simulink model "task_2_sim"  (R2023a)
settings: Solver=VariableStepAuto  StartTime=0.0  StopTime=6  MaxStep=1e-4  RelTol=1e-4
undefined symbols (not defined in the file): Ab, Bb, Cb, Cz, D, Dz, Kb, L, xw0, Y1, Y2, Yg
settings Model: Creator=user  LastModifiedBy=user

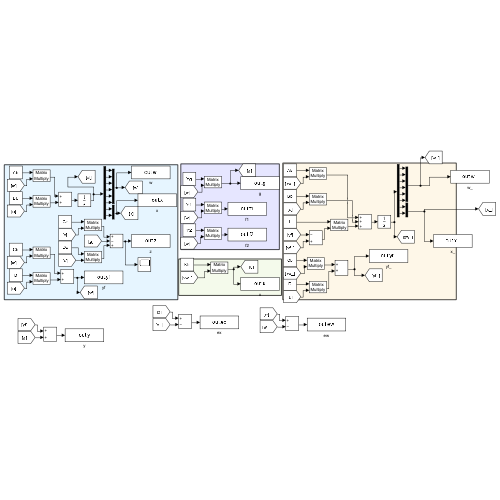
[thumbnail: Simulink's stored preview of the top-level diagram]
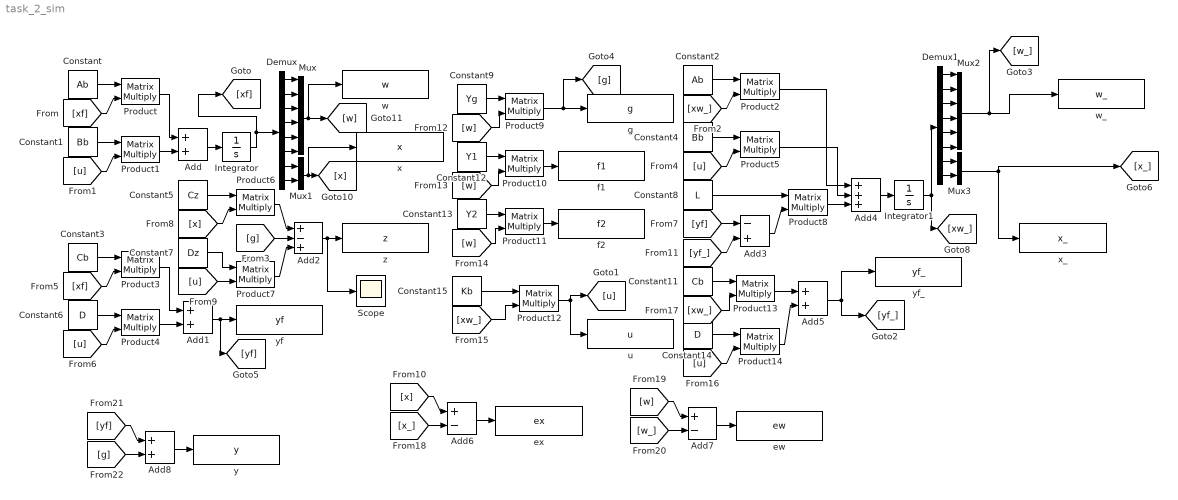
== system task_2_sim ==
  Add{,1,5,8} (4 alike) : Sum
  Add2 : Sum  Inputs=+-+
  Add3 : Sum  Inputs=-+
  Add4 : Sum  Inputs=+++
  Add6 : Sum  Inputs=+-
  Add7 : Sum  Inputs=+-
  Constant : Constant  Value=Ab  VectorParams1D=off
  Constant1 : Constant  Value=Bb  VectorParams1D=off
  Constant11 : Constant  Value=Cb  VectorParams1D=off
  Constant12 : Constant  Value=Y1  VectorParams1D=off
  Constant13 : Constant  Value=Y2  VectorParams1D=off
  Constant14 : Constant  Value=D  VectorParams1D=off
  Constant15 : Constant  Value=Kb  VectorParams1D=off
  Constant2 : Constant  Value=Ab  VectorParams1D=off
  Constant3 : Constant  Value=Cb  VectorParams1D=off
  Constant4 : Constant  Value=Bb  VectorParams1D=off
  Constant5 : Constant  Value=Cz  VectorParams1D=off
  Constant6 : Constant  Value=D  VectorParams1D=off
  Constant7 : Constant  Value=Dz  VectorParams1D=off
  Constant8 : Constant  Value=L  VectorParams1D=off
  Constant9 : Constant  Value=Yg  VectorParams1D=off
  Demux : Demux  Outputs=8
  Demux1 : Demux  Outputs=8
  Integrator : Integrator  InitialCondition=xw0
  Integrator1 : Integrator
  Mux : Mux  Inputs=6
  Mux1 : Mux  Inputs=2
  Mux2 : Mux  Inputs=6
  Mux3 : Mux  Inputs=2
  Product{,1..14} (15 alike) : Product  Multiplication=Matrix(*)
  Scope : Scope
  ew : ToWorkspace  VariableName=ew  SaveFormat=Timeseries  SampleTime=-1
  ex : ToWorkspace  VariableName=ex  SaveFormat=Timeseries  SampleTime=-1
  f1 : ToWorkspace  VariableName=f1  SaveFormat=Timeseries  SampleTime=-1
  f2 : ToWorkspace  VariableName=f2  SaveFormat=Timeseries  SampleTime=-1
  g : ToWorkspace  VariableName=g  SaveFormat=Timeseries  SampleTime=-1
  u : ToWorkspace  VariableName=u  SaveFormat=Timeseries  SampleTime=-1
  w : ToWorkspace  VariableName=w  SaveFormat=Timeseries  SampleTime=-1
  w_ : ToWorkspace  VariableName=w_  SaveFormat=Timeseries  SampleTime=-1
  x : ToWorkspace  VariableName=x  SaveFormat=Timeseries  SampleTime=-1
  x_ : ToWorkspace  VariableName=x_  SaveFormat=Timeseries  SampleTime=-1
  y : ToWorkspace  VariableName=y  SaveFormat=Timeseries  SampleTime=-1
  yf : ToWorkspace  VariableName=yf  SaveFormat=Timeseries  SampleTime=-1
  yf_ : ToWorkspace  VariableName=yf_  SaveFormat=Timeseries  SampleTime=-1
  z : ToWorkspace  VariableName=z  SaveFormat=Timeseries  SampleTime=-1
  wires:
  Constant/1 -> Product/1
  [xf] -> Product/2
  Constant1/1 -> Product1/1
  [u] -> Product1/2
  Constant3/1 -> Product3/1
  [xf] -> Product3/2
  Constant6/1 -> Product4/1
  [u] -> Product4/2
  Product4/1 -> Add1/2
  Product1/1 -> Add/2
  Product3/1 -> Add1/1
  Product/1 -> Add/1
  Add/1 -> Integrator/1
  Integrator/1 -> Demux/1, [xf]
  Add1/1 -> [yf], yf/1
  Constant5/1 -> Product6/1
  [x] -> Product6/2
  [u] -> Product7/2
  Constant7/1 -> Product7/1
  [g] -> Add2/2
  Product7/1 -> Add2/3
  Product6/1 -> Add2/1
  Add2/1 -> Scope/1, z/1
  Constant9/1 -> Product9/1
  [w] -> Product9/2
  Product9/1 -> g/1, [g]
  [w] -> Product10/2
  Constant12/1 -> Product10/1
  Product10/1 -> f1/1
  Constant13/1 -> Product11/1
  [w] -> Product11/2
  Product11/1 -> f2/1
  Constant15/1 -> Product12/1
  [xw_] -> Product12/2
  Product12/1 -> u/1, [u]
  Demux/1 -> Mux/1
  Demux/2 -> Mux/2
  Demux/3 -> Mux/3
  Demux/4 -> Mux/4
  Demux/5 -> Mux/5
  Demux/6 -> Mux/6
  Demux/7 -> Mux1/1
  Demux/8 -> Mux1/2
  Mux1/1 -> x/1, [x]
  Mux/1 -> w/1, [w]
  Constant2/1 -> Product2/1
  [xw_] -> Product2/2
  Constant4/1 -> Product5/1
  [u] -> Product5/2
  [yf_] -> Add3/2
  [yf] -> Add3/1
  Constant8/1 -> Product8/1
  Add3/1 -> Product8/2
  Product8/1 -> Add4/3
  Product5/1 -> Add4/2
  Product2/1 -> Add4/1
  [xw_] -> Product13/2
  Constant11/1 -> Product13/1
  [u] -> Product14/2
  Constant14/1 -> Product14/1
  Product13/1 -> Add5/1
  Product14/1 -> Add5/2
  Add5/1 -> [yf_], yf_/1
  Mux3/1 -> x_/1, [x_]
  Demux1/7 -> Mux3/1
  Demux1/2 -> Mux2/2
  Demux1/4 -> Mux2/4
  Demux1/5 -> Mux2/5
  Demux1/3 -> Mux2/3
  Mux2/1 -> [w_], w_/1
  Demux1/6 -> Mux2/6
  Demux1/8 -> Mux3/2
  Demux1/1 -> Mux2/1
  Add4/1 -> Integrator1/1
  Integrator1/1 -> [xw_], Demux1/1
  [x_] -> Add6/2
  [x] -> Add6/1
  Add6/1 -> ex/1
  [w] -> Add7/1
  Add7/1 -> ew/1
  [w_] -> Add7/2
  [yf] -> Add8/1
  Add8/1 -> y/1
  [g] -> Add8/2
